simulink library "MSP_env_estim"  (R2016b)
settings: Solver=VariableStepAuto  StartTime=0.0  StopTime=10.0  RelTol=1e-3
undefined symbols (not defined in the file or in its folder): fsw_params
libraries: time_conversion_lib x1, gs_prediction_lib x1, mag_vec_LS_lib x1, mag_vec_lib x1, sgp4_lib_fsw x1, sun_vector_lib x1, time_coord_rotation_lib x1
settings Model: Creator=taylorreynolds  LastModifiedBy=taylorreynolds

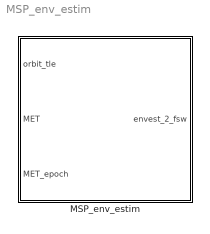
== system MSP_env_estim ==
  MSP_env_estim : Subsystem

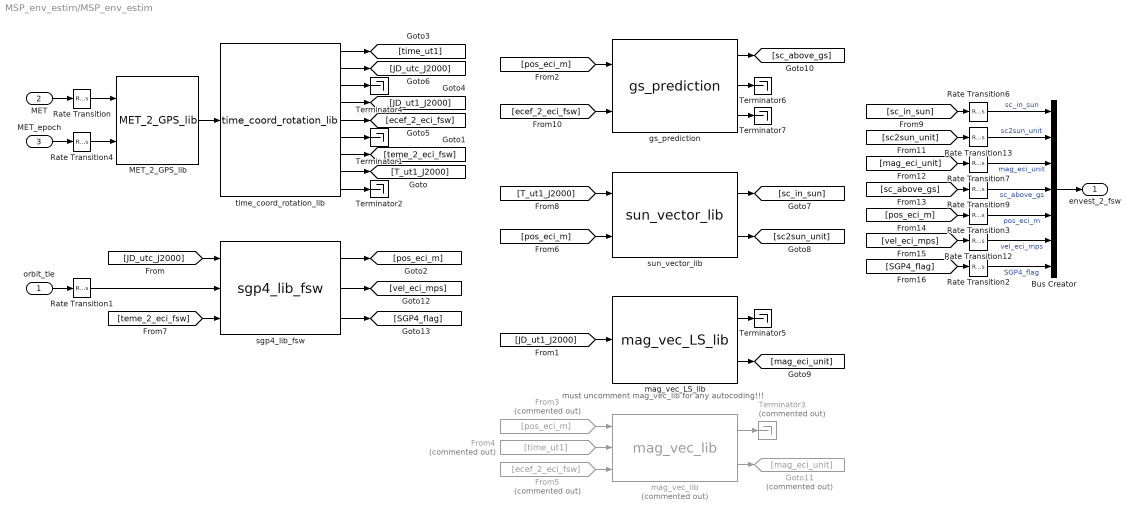
== system MSP_env_estim/MSP_env_estim ==
  note: must uncomment mag_vec_lib for any autocoding!!!
  orbit_tle : Inport
  MET : Inport  Port=2
  MET_epoch : Inport  Port=3
  Bus Creator : BusCreator  Inputs=7
  From3 : From  Commented=on  GotoTag=pos_eci_m
  From4 : From  Commented=on  GotoTag=time_ut1
  From5 : From  Commented=on  GotoTag=ecef_2_eci_fsw
  Goto11 : Goto  Commented=on  GotoTag=mag_eci_unit
  MET_2_GPS_lib : time_conversion_lib/MET_2_GPS_lib
  Rate Transition : RateTransition  OutPortSampleTime=fsw_params.env_estimation.sample_time_s
  Rate Transition1 : RateTransition  X0=fsw_params.env_estimation.ic.orbit_tle  OutPortSampleTime=fsw_params.env_estimation.sample_time_s
  Rate Transition{2..3,6..7,9,12..13} (7 alike) : RateTransition
  Rate Transition4 : RateTransition  X0=fsw_params.constants.ic.time.JD_J2000_TT_s  OutPortSampleTime=fsw_params.env_estimation.sample_time_s
  Terminator{1..2,4..7} (6 alike) : Terminator
  Terminator3 : Terminator  Commented=on
  gs_prediction : gs_prediction_lib/gs_prediction
  mag_vec_LS_lib : mag_vec_LS_lib/mag_vec_LS_lib
  mag_vec_lib : mag_vec_lib/mag_vec_lib  Commented=on
  sgp4_lib_fsw : sgp4_lib_fsw/sgp4_lib_fsw
  sun_vector_lib : sun_vector_lib/sun_vector_lib
  time_coord_rotation_lib : time_coord_rotation_lib/time_coord_rotation_lib
  envest_2_fsw : Outport
  wires:
  mag_vec_LS_lib/2 -> [mag_eci_unit]
  sun_vector_lib/2 -> [sc2sun_unit]
  [T_ut1_J2000] -> sun_vector_lib/1
  [JD_utc_J2000] -> sgp4_lib_fsw/1
  sun_vector_lib/1 -> [sc_in_sun]
  [pos_eci_m] -> sun_vector_lib/2
  sgp4_lib_fsw/1 -> [pos_eci_m]
  orbit_tle/1 -> Rate Transition1/1
  MET/1 -> Rate Transition/1
  time_coord_rotation_lib/1 -> [time_ut1]
  gs_prediction/1 -> [sc_above_gs]
  Rate Transition1/1 -> sgp4_lib_fsw/2
  gs_prediction/2 -> Terminator6/1
  gs_prediction/3 -> Terminator7/1
  Rate Transition6/1 -> Bus Creator/1  "sc_in_sun"
  mag_vec_LS_lib/1 -> Terminator5/1
  [ecef_2_eci_fsw] -> gs_prediction/2
  [pos_eci_m] -> gs_prediction/1
  time_coord_rotation_lib/9 -> Terminator2/1
  time_coord_rotation_lib/8 -> [T_ut1_J2000]
  time_coord_rotation_lib/7 -> [teme_2_eci_fsw]
  time_coord_rotation_lib/6 -> Terminator1/1
  time_coord_rotation_lib/5 -> [ecef_2_eci_fsw]
  time_coord_rotation_lib/4 -> [JD_ut1_J2000]
  time_coord_rotation_lib/3 -> Terminator4/1
  time_coord_rotation_lib/2 -> [JD_utc_J2000]
  [teme_2_eci_fsw] -> sgp4_lib_fsw/3
  sgp4_lib_fsw/2 -> [vel_eci_mps]
  sgp4_lib_fsw/3 -> [SGP4_flag]
  Rate Transition/1 -> MET_2_GPS_lib/1
  MET_2_GPS_lib/1 -> time_coord_rotation_lib/1
  [JD_ut1_J2000] -> mag_vec_LS_lib/1
  mag_vec_lib/2 -> Goto11/1
  From3/1 -> mag_vec_lib/1
  From4/1 -> mag_vec_lib/2
  From5/1 -> mag_vec_lib/3
  mag_vec_lib/1 -> Terminator3/1
  [sc_in_sun] -> Rate Transition6/1
  [sc2sun_unit] -> Rate Transition13/1
  Rate Transition13/1 -> Bus Creator/2  "sc2sun_unit"
  Rate Transition7/1 -> Bus Creator/3  "mag_eci_unit"
  [mag_eci_unit] -> Rate Transition7/1
  Rate Transition9/1 -> Bus Creator/4  "sc_above_gs"
  [sc_above_gs] -> Rate Transition9/1
  Rate Transition3/1 -> Bus Creator/5  "pos_eci_m"
  [pos_eci_m] -> Rate Transition3/1
  Rate Transition12/1 -> Bus Creator/6  "vel_eci_mps"
  [vel_eci_mps] -> Rate Transition12/1
  Rate Transition2/1 -> Bus Creator/7  "SGP4_flag"
  [SGP4_flag] -> Rate Transition2/1
  Bus Creator/1 -> envest_2_fsw/1
  MET_epoch/1 -> Rate Transition4/1
  Rate Transition4/1 -> MET_2_GPS_lib/2
